simulink model "modelloSatelliteSottoattuato"  (R2025b)
settings: Solver=VariableStepAuto  StartTime=0.0  StopTime=10  RelTol=1e-3
values from neighbouring files (symbols this model uses):
  I = [13470; 20450; 27200]    [main.m]
  K = diag([20 20 20])    [main.m]
settings Model: Creator=Armando  LastModifiedBy=Armando

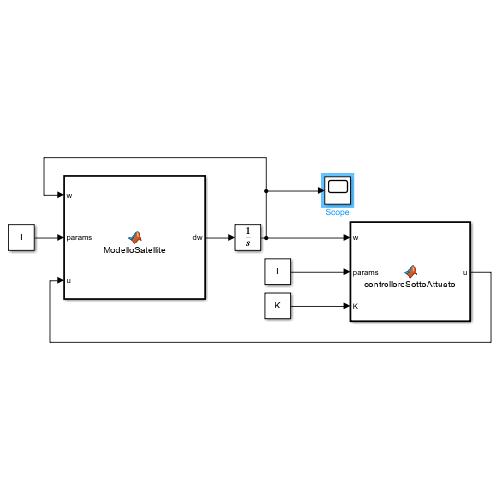
[thumbnail: Simulink's stored preview of the top-level diagram]
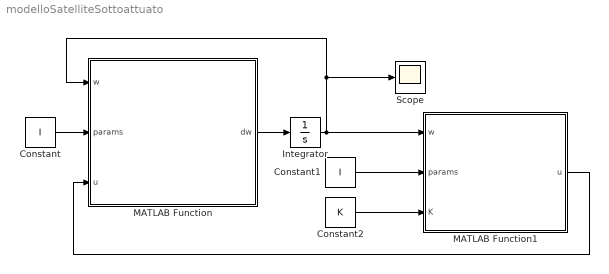
== system modelloSatelliteSottoattuato ==
  Constant : Constant  Value=I  VectorParams1D=off
  Constant1 : Constant  Value=I  VectorParams1D=off
  Constant2 : Constant  Value=K
  Integrator : Integrator  InitialCondition=[1;1;1]
  MATLAB Function : MATLAB Function  TreatAsAtomicUnit=on
  MATLAB Function1 : MATLAB Function  TreatAsAtomicUnit=on
  Scope : Scope
      settings: ActiveDisplayYMinimum=-0.1629632130145815  ActiveDisplayYMaximum=34.965500286814304
  wires:
  MATLAB Function/1(dw) -> Integrator/1
  Integrator/1 -> Scope/1, MATLAB Function/1(w), MATLAB Function1/1(w)
  Constant/1 -> MATLAB Function/2(params)
  Constant1/1 -> MATLAB Function1/2(params)
  Constant2/1 -> MATLAB Function1/3(K)
  MATLAB Function1/1(u) -> MATLAB Function/3(u)

== matlab function modelloSatelliteSottoattuato/MATLAB Function ==
  data: w input; params input; u input; dw output
function dw = ModelloSatellite(w,params,u)
    c = [(params(2) - params(3))/params(1)*w(2)*w(3);
         ( params(3)- params(1))/params(2)*w(3)*w(1);
          (params(1) - params(2))/params(3)*w(1)*w(2)];
    
    dw = c + (u./params(:));

== matlab function modelloSatelliteSottoattuato/MATLAB Function1 ==
  data: w input; params input; u output; K input
function u = controlloreSottoAttuato(w,params,K)

    I1 = params(1); I2 = params(2); I3 = params(3);

    lambda = 0.5;

    c  = (I1-I2)/I3;
    k  = K(3,3); k1 = K(1,1); k2 = K(2,2);
    
    %riferimenti virtuali
    w1_star = lambda*w(3); w2_star = -(k/(c*lambda))*w(3)^2;

    wdot3 = c*w(1)*w(2);
    
    w1_tilde = w(1) - w1_star;
    w2_tilde = w(2) - w2_star;

   % Controlli
    u1 = I1*lambda*wdot3 - (I2-I3)*(-k/(c*lambda)*w(3)^2 + w2_tilde)*w(3) - I1*k1*w1_tilde;
    
    u2 = -(2*k*I2/(c*lambda))*w(3)*wdot3 - (I3-I1)*(lambda*w(3) + w1_tilde)*w(3)- I2*k2*w2_tilde;

    % Sistema sottoattuato: il terzo ingresso non è disponibile
    u = [u1; u2; 0];
